simulink model "bfsk"  (R2019a)
settings: Solver=VariableStepAuto  StartTime=0.0  StopTime=10.0  RelTol=1e-3
settings Model: Creator=dante  LastModifiedBy=dante

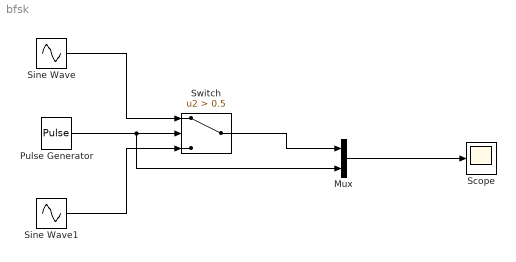
== system bfsk ==
  Mux : Mux  Inputs=2
  Pulse Generator : DiscretePulseGenerator  PulseType=Time based  PulseWidth=50
  Scope : Scope
  Sine Wave : Sin  Frequency=30  SampleTime=0.0001
  Sine Wave1 : Sin  Frequency=10  SampleTime=0.0001
  Switch : Switch  Criteria=u2 > Threshold  Threshold=0.5
  wires:
  Sine Wave/1 -> Switch/1
  Sine Wave1/1 -> Switch/3
  Pulse Generator/1 -> Mux/2, Switch/2
  Switch/1 -> Mux/1
  Mux/1 -> Scope/1
